simulink model "HW4_PID_adarbha"  (Simulink 7.7)
settings: Solver=ode45  StartTime=0.0  StopTime=max(time_s)  RelTol=1e-3
values from neighbouring files (symbols this model uses):
  Area = 2.7    [adarbha_drivecycle.m]
  Cd = 0.44    [adarbha_drivecycle.m]
  density = 1.224    [adarbha_drivecycle.m]
  rpm = 1:5000    [adarbha_drivecycle.m]
  time_s = time_scale*100    [adarbha_drivecycle.m]
  vel_m_s = M_number*3    [adarbha_drivecycle.m]
  weight_N = 16000    [adarbha_drivecycle.m]
undefined symbols (not defined in the file or in its folder): torque
libraries: simulink x1
settings Model: Creator=Arjun  LastModifiedBy=Arjun

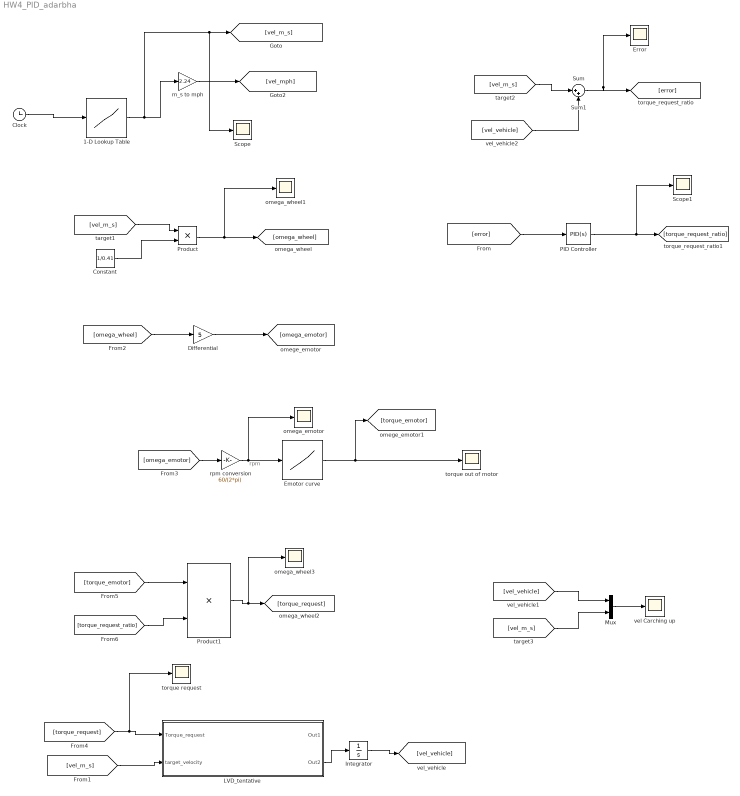
== system HW4_PID_adarbha ==
  note: rpm
  1-D Lookup Table : Lookup_n-D  NumberOfTableDimensions=1  BreakpointsForDimension1=time_s  Table=vel_m_s  RndMeth=Simplest  InputSameDT=on
  Clock : Clock
      settings: Decimation=10
  Constant : Constant  Value=1/0.41
  Differential : Gain  Gain=5
  Emotor curve : Lookup_n-D  NumberOfTableDimensions=1  BreakpointsForDimension1=rpm  Table=torque  RndMeth=Simplest  InputSameDT=on
  Error : Scope
  Integrator : Integrator
  LVD_tentative : Subsystem
  Mux : Mux  Inputs=2
  PID Controller : simulink/Continuous/PID Controller  SystemSampleTime=-1  Controller=PID  TimeDomain=Continuous-time  SampleTime=1  IntegratorMethod=Forward Euler  FilterMethod=Forward Euler  Form=Parallel  P=1.18584226429726  I=0.0109103789645266  D=-0.533451149274748  N=2.22296318211981  InitialConditionSource=internal  InitialConditionForIntegrator=0  InitialConditionForFilter=0  ExternalReset=none  LimitOutput=off  UpperSaturationLimit=inf  LowerSaturationLimit=-inf  LinearizeAsGain=off  AntiWindupMode=none  Kb=1  TrackingMode=off  Kt=1  PParamMin=[]  PParamMax=[]  IParamMin=[]  IParamMax=[]  DParamMin=[]  DParamMax=[]  NParamMin=[]  NParamMax=[]  KbParamMin=[]  KbParamMax=[]  KtParamMin=[]  KtParamMax=[]  POutMin=[]  POutMax=[]  IOutMin=[]  IOutMax=[]  DOutMin=[]  DOutMax=[]  NOutMin=[]  NOutMax=[]  KbOutMin=[]  KbOutMax=[]  KtOutMin=[]  KtOutMax=[]  IntegratorOutMin=[]  IntegratorOutMax=[]  FilterOutMin=[]  FilterOutMax=[]  SumOutMin=[]  SumOutMax=[]  SumI1OutMin=[]  SumI1OutMax=[]  SumI2OutMin=[]  SumI2OutMax=[]  SumI3OutMin=[]  SumI3OutMax=[]  SumDOutMin=[]  SumDOutMax=[]  SaturationOutMin=[]  SaturationOutMax=[]  IntegratorContinuousStateAttributes=''  IntegratorStateMustResolveToSignalObject=off  IntegratorRTWStateStorageClass=Auto  FilterContinuousStateAttributes=''  FilterStateMustResolveToSignalObject=off  FilterRTWStateStorageClass=Auto
  Product : Product  RndMeth=Zero
  Product1 : Product  RndMeth=Zero
  Scope : Scope
  Scope1 : Scope
      settings: SaveName=ScopeData2
  Sum : Sum  Inputs=|+-
  Sum1 : Sum  Inputs=|++
  m_s to mph : Gain  Gain=2.24
  omega_emotor : Scope
      settings: SaveName=ScopeData4
  omega_wheel1 : Scope
      settings: SaveName=ScopeData3
  omega_wheel3 : Scope
      settings: SaveName=ScopeData6
  rpm conversion : Gain  Gain=60/(2*pi)
  torque out of motor : Scope
      settings: SaveName=ScopeData5
  torque request : Scope
      settings: SaveName=ScopeData11
  vel Carching up : Scope
      settings: SaveName=ScopeData7
  wires:
  1-D Lookup Table/1 -> m_s to mph/1, [vel_m_s], Scope/1
  m_s to mph/1 -> [vel_mph]
  Clock/1 -> 1-D Lookup Table/1
  [vel_m_s] -> Sum/1
  [vel_vehicle] -> Sum/2
  Sum/1 -> Error/1, [error]
  [error] -> PID Controller/1
  PID Controller/1 -> [torque_request_ratio], Scope1/1
  [vel_m_s] -> Product/1
  Product/1 -> [omega_wheel], omega_wheel1/1
  Constant/1 -> Product/2
  [omega_wheel] -> Differential/1
  Differential/1 -> [omega_emotor]
  [omega_emotor] -> rpm conversion/1
  rpm conversion/1 -> Emotor curve/1, omega_emotor/1
  Emotor curve/1 -> torque out of motor/1, [torque_emotor]
  [torque_emotor] -> Product1/1
  [torque_request_ratio] -> Product1/2
  Product1/1 -> [torque_request], omega_wheel3/1
  [vel_m_s] -> LVD_tentative/2(target_velocity)
  [torque_request] -> LVD_tentative/1(Torque_request), torque request/1
  Integrator/1 -> [vel_vehicle]
  LVD_tentative/2(Out2) -> Integrator/1
  [vel_m_s] -> Mux/2
  Mux/1 -> vel Carching up/1
  [vel_vehicle] -> Mux/1

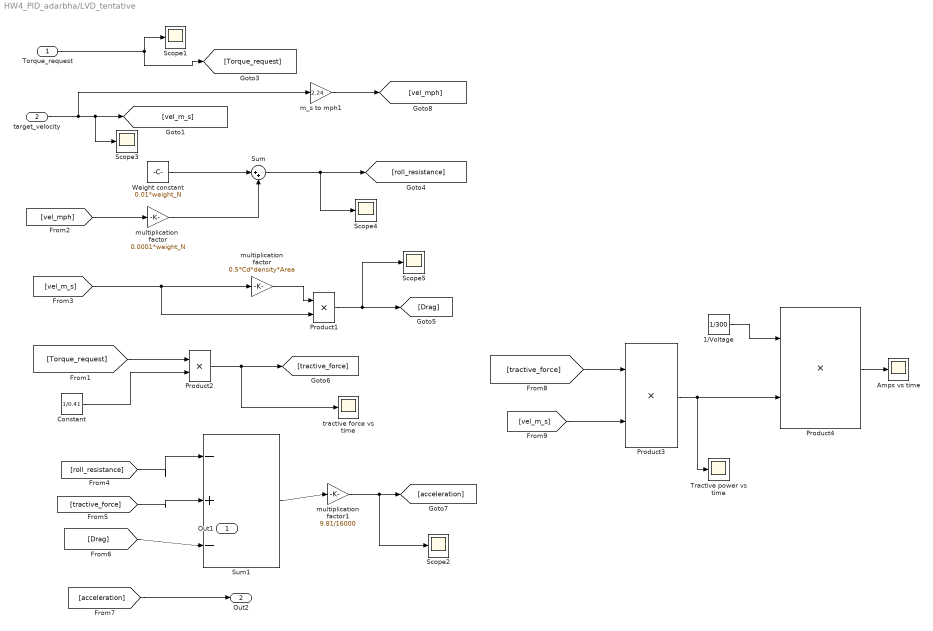
== system HW4_PID_adarbha/LVD_tentative ==
  Torque_request : Inport
  target_velocity : Inport  Port=2
  1/Voltage : Constant  Value=1/300
  Amps vs time : Scope
      settings: SaveName=ScopeData15
  Constant : Constant  Value=1/0.41
  Product{1..4} (4 alike) : Product  RndMeth=Zero
  Scope{1..5} (5 alike) : Scope
      Scope1 settings: SaveName=ScopeData5
      Scope2 settings: SaveName=ScopeData6
      Scope3 settings: SaveName=ScopeData8
      Scope4 settings: SaveName=ScopeData9
      Scope5 settings: SaveName=ScopeData10
  Sum : Sum  Inputs=|++
  Sum1 : Sum  Inputs=|-+-
  Tractive power vs time : Scope
      settings: SaveName=ScopeData14
  Weight constant : Constant  Value=0.01*weight_N
  m_s to mph1 : Gain  Gain=2.24
  multiplication  factor : Gain  Gain=0.0001*weight_N
  multiplication factor : Gain  Gain=0.5*Cd*density*Area
  multiplication factor1 : Gain  Gain=9.81/16000
  tractive force vs time : Scope
      settings: SaveName=ScopeData13
  Out1 : Outport
  Out2 : Outport  Port=2
  wires:
  Weight constant/1 -> Sum/1
  multiplication  factor/1 -> Sum/2
  Sum/1 -> [roll_resistance], Scope4/1
  [vel_mph] -> multiplication  factor/1
  multiplication factor/1 -> Product1/1
  [vel_m_s] -> multiplication factor/1, Product1/2
  Product1/1 -> [Drag], Scope5/1
  [Torque_request] -> Product2/1
  Constant/1 -> Product2/2
  Product2/1 -> [tractive_force], tractive force vs time/1
  [roll_resistance] -> Sum1/1
  [tractive_force] -> Sum1/2
  [Drag] -> Sum1/3
  Sum1/1 -> multiplication factor1/1
  multiplication factor1/1 -> [acceleration], Scope2/1
  Torque_request/1 -> [Torque_request], Scope1/1
  target_velocity/1 -> m_s to mph1/1, [vel_m_s], Scope3/1
  m_s to mph1/1 -> [vel_mph]
  [acceleration] -> Out2/1
  [tractive_force] -> Product3/1
  [vel_m_s] -> Product3/2
  Product3/1 -> Tractive power vs time/1, Product4/2
  1/Voltage/1 -> Product4/1
  Product4/1 -> Amps vs time/1
